simulink model "Crane_rigid"  (R2021b)
settings: Solver=ode15s  StartTime=0.0  StopTime=t_f  MaxStep=max_step_size  RelTol=1e-3
values from neighbouring files (symbols this model uses):
  a_d_full_y = circshift(a_d_full_x,floor(1/h))/2    [modify_tracking.m]
  cont_param_10 = in    [double_pendulum.m]    (also in optimize_10_SMC_single_first_explicit.m = cont_param_10_surrogateopt)
  cont_param_11 = in    [double_pendulum.m]    (also in optimize_11_SMC_single_first_implicit.m = cont_param_11_surrogateopt)
  cont_param_12 = in    [double_pendulum.m]    (also in optimize_12_SMC_single_last_explicit.m = cont_param_12_surrogateopt)
  cont_param_13 = in    [double_pendulum.m]    (also in optimize_13_SMC_single_last_implicit.m = cont_param_13_surrogateopt)
  cont_param_14 = in    [double_pendulum.m]    (also in optimize_14_SMC_double_explicit.m = cont_param_14_surrogateopt)
  cont_param_15 = in    [double_pendulum.m]    (also in optimize_15_SMC_double_implicit.m = cont_param_15_surrogateopt)
  cont_param_16 = in    [double_pendulum.m]
  cont_param_17 = in    [double_pendulum.m]
  cont_param_18 = in    [double_pendulum.m]
  cont_param_19 = in    [double_pendulum.m]
  cont_param_4 = in    [double_pendulum.m]
  cont_param_5 = in    [double_pendulum.m]
  cont_param_6 = in    [double_pendulum.m]
  cont_param_7 = in    [double_pendulum.m]
  cont_param_8 = in    [double_pendulum.m]
  cont_param_9 = in    [double_pendulum.m]
  h = 1e-5    (= 1e-05)    [Conference_paper.m]    (also in Latest.m)
  m = 10    [Conference_paper.m]    (also in Latest.m = 100; control_8_collocated_PD_tracking.m = load_mass+hook_mass+cable_mass_total)
  method_select = Method    [main_run.m]    (also in modify_tracking.m = 3)
  N = floor(t_f / h)    [control_2_zero_vibration.m]    (also in control_3_ZVD.m; modify_tracking.m = 3)
  s = c1*(x-xd)+c2*(v-vd)+c3*theta_dot_1+c4*theta_1    [control_10_SMC_single_first_explicit.m]    (also in control_11_SMC_single_first_implicit.m = c1*(x-xd)+c2*(v-vd)+c3*theta_dot+c4*theta; control_12_SMC_single_last_explicit.m = c1*(x-xd)+c2*(v-vd)+c3*theta_dot_2+c4*theta_2; control_13_SMC_single_last_implicit.m = c1*(x-xd)+c2*(v-vd)+c3*theta_dot+c4*theta; control_14_SMC_double_explicit.m = (v-vd)+lambda*(x-xd)+alpha*theta_1+beta*theta_2)
  sin_traj_w = 0.5    [modify_tracking.m]
  X = ex+lambda*sin(theta)    [control_16_PD_energy_first.m]    (also in control_17_PD_energy_last.m)
  Z = cont_param_8(4)    [control_8_collocated_PD_tracking.m]
undefined symbols (not defined in the file or in its folder): a_d_full_x, all_initial_sway, c_actuator, cable_length, cable_mass_total, cart_disturbance_amp, cart_mass, delay_time, first_link_sway, hook_mass, last_piece_length, load_disturbance_amp, number_of_pendulums, payload_mass, sat_const, sin_traj_A, t_f, total_mass, traj_number, unbalanced_factor, Y
libraries: nesl_utility x180, sm_lib x138, commchan3 x8
(part 1 of 3)
settings Model: Creator=rmoja  LastModifiedBy=SESA642626

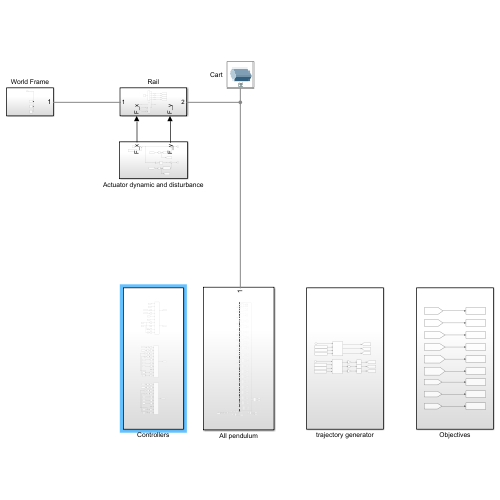
[thumbnail: Simulink's stored preview of the top-level diagram]
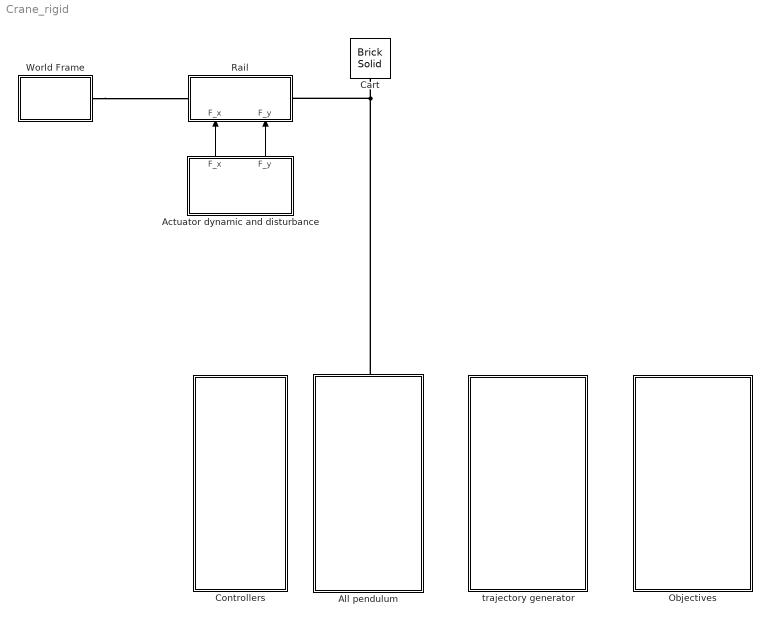
== system Crane_rigid ==
  Actuator dynamic and disturbance : Subsystem
  All pendulum : Subsystem
      settings: PortSchema="{\"entries\":[{\"content\":{\"sides\":[{\"content\":{\"connectorIds\":[]},\"type\":\"ConnectorPlacement.EquallySpacedRectSide\",\"uuid\":\"a0695cec-8b60-4481-8da3-91054655feca\"},{\"content\":{\"connectorIds\":[],\"side\":\"RIGHT\"},\"type\":\"ConnectorPlacement.EquallySpacedRectSide\",\"uuid\":\"63fc90b5-61bb-43b2-b1de-87e85d16d1ba\"},{\"content\":{\"connectorIds\":[\"LConn1\"],\"side\":\"TOP\"},\"type\":\"ConnectorPlacement.EquallySpacedRectSide\",\"uuid\":\"b1a79959-5d9b-4237-a357-9ee6cf3ddb2d\"}]},\"type\":\"ConnectorPlacement.EquallySpacedConnector\",\"uuid\":\"2998d234-7b55-409a-8879-2241677dc568\"}],\"packageUris\":[\"http://schema.mathworks.com/mf0/Connector/R2020b\"],\"version\":\"1.0\"}"
  Cart : sm_lib/Body Elements/Brick Solid  GraphicAmbientColor=[0.15 0.15 0.15 1.0]  BasedOnType=Mass  BrickDimensions=[1 1 1]  BrickDimensionUnits=m  CenterOfMass=[0 0 0]  CenterOfMassUnits=m  GraphicDiffuseColor=[0.8 0.0 0.8]  Density=1000  DensityUnits=kg/(m^3)  DoExposeReferenceFrame=on  GraphicEmissiveColor=[0.0 0.0 0.0 1.0]  ExportEntireGeometry=off  SerializedFrames=<Frames/>  MarkerShape=Sphere  MarkerSize=10  GraphicType=FromGeometry  InertiaType=PointMass  Mass=cart_mass  MassUnits=kg  MomentsOfInertia=[1 1 1]  MomentsOfInertiaUnits=kg*m^2  GraphicOpacity=1.0  ProductsOfInertia=[0 0 0]  ProductsOfInertiaUnits=kg*m^2  GraphicShininess=75  GraphicSpecularColor=[0.5 0.5 0.5 1.0]  GraphicVisPropType=SimpleVisualProperties
  Controllers : Subsystem
  Objectives : Subsystem
  Rail : Subsystem
      settings: PortSchema="{\"entries\":[{\"content\":{\"sides\":[{\"content\":{\"connectorIds\":[\"LConn1\"]},\"type\":\"ConnectorPlacement.EquallySpacedRectSide\",\"uuid\":\"d9e65a69-c05e-4610-81fe-2f9f88514456\"},{\"content\":{\"connectorIds\":[\"RConn1\"],\"side\":\"RIGHT\"},\"type\":\"ConnectorPlacement.EquallySpacedRectSide\",\"uuid\":\"de9124b5-abd7-4a44-8ac0-9f1bb82b9c20\"},{\"content\":{\"connectorIds\":[],\"side\":\"TOP\"},\"type\":\"ConnectorPlacement.EquallySpacedRectSide\",\"uuid\":\"433c8926-32eb-4eac-9405-2f674875eeab\"},{\"content\":{\"connectorIds\":[\"In1\",\"In2\"],\"side\":\"BOTTOM\"},\"type\":\"ConnectorPlacement.EquallySpacedRectSide\",\"uuid\":\"d2188721-54bd-44ea-91c1-f694293db46f\"}]},\"type\":\"ConnectorPlacement.EquallySpacedConnector\",\"uuid\":\"441db2e5-934f-48d0-8bd6-b56c902c81c4\"}],\"packageUris\":[\"http://schema.mathworks.com/mf0/Connector/R2020b\"],\"version\":\"1.0\"}"
  World Frame : Subsystem
  trajectory generator : Subsystem
  wires:
  Actuator dynamic and disturbance/1(F_x) -> Rail/1(F_x)
  Actuator dynamic and disturbance/2(F_y) -> Rail/2(F_y)
  connections:
  World Frame/LConn1 -- Rail/LConn1
  All pendulum/LConn1 -- Rail/RConn1 -- Cart/RConn1

== system Crane_rigid/Actuator dynamic and disturbance ==
  Actuator : TransferFcn  Numerator=[c_actuator]  Denominator=[1 c_actuator]
  Actuator1 : TransferFcn  Numerator=[c_actuator]  Denominator=[1 c_actuator]
  Constant : Constant  Value=cart_disturbance_amp
  Gain : Gain  Gain=0.5
  Pulse Generator : DiscretePulseGenerator  PulseType=Time based  Amplitude=2*cart_disturbance_amp  Period=20  PulseWidth=50
  Saturation1 : Saturate  UpperLimit=+sat_const  LowerLimit=-sat_const
  Saturation2 : Saturate  UpperLimit=+sat_const  LowerLimit=-sat_const
  Sum : Sum  Inputs=|+-
  Sum1 : Sum  Inputs=|++
  Sum3 : Sum  Inputs=|++
  Transport Delay : TransportDelay
  F_x : Outport
  F_y : Outport  Port=2
  tag scope: F_x_after_sat=global, F_y_after_sat=global
  wires:
  Actuator/1 -> Sum1/2
  Sum1/1 -> F_x/1
  Saturation1/1 -> [F_x_after_sat], Actuator/1
  [Control_output_x] -> Saturation1/1
  Sum3/1 -> F_y/1
  [Control_output_y] -> Saturation2/1
  Saturation2/1 -> [F_y_after_sat], Actuator1/1
  Actuator1/1 -> Sum3/2
  Pulse Generator/1 -> Sum/1
  Constant/1 -> Sum/2
  Sum/1 -> Gain/1, Sum1/1
  Gain/1 -> Transport Delay/1
  Transport Delay/1 -> Sum3/1  "yd"

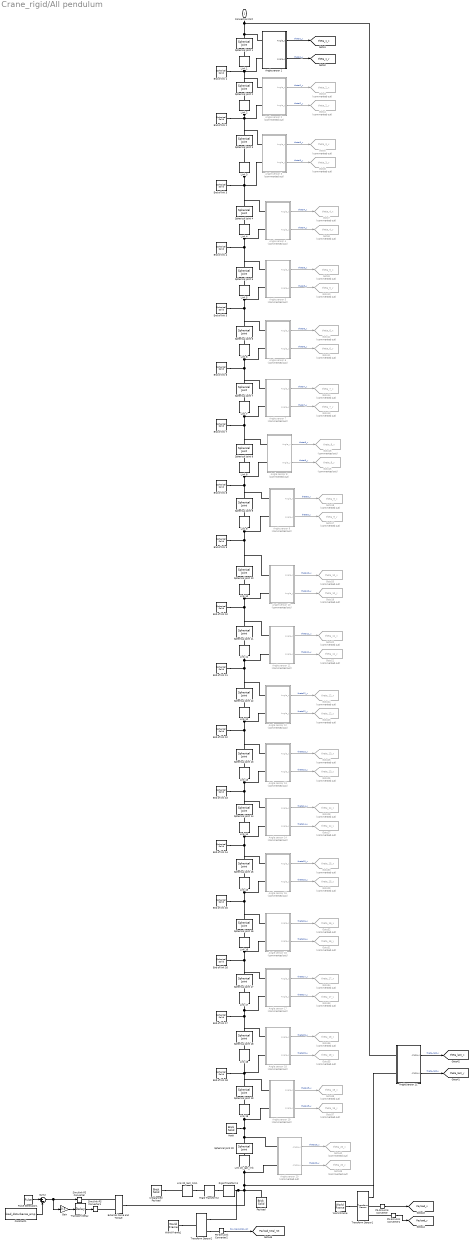
== system Crane_rigid/All pendulum ==
  Angle sensor 1 : Subsystem
  Angle sensor 10 : Subsystem  Commented=on
  Angle sensor 11 : Subsystem  Commented=on
  Angle sensor 12 : Subsystem  Commented=on
  Angle sensor 13 : Subsystem  Commented=on
  Angle sensor 14 : Subsystem  Commented=on
  Angle sensor 15 : Subsystem  Commented=on
  Angle sensor 16 : Subsystem  Commented=on
  Angle sensor 17 : Subsystem  Commented=on
  Angle sensor 18 : Subsystem  Commented=on
  Angle sensor 19 : Subsystem  Commented=on
  Angle sensor 2 : Subsystem  Commented=on
  Angle sensor 20 : Subsystem  Commented=on
  Angle sensor 21 : Subsystem
  Angle sensor 3 : Subsystem  Commented=on
  Angle sensor 4 : Subsystem  Commented=on
  Angle sensor 5 : Subsystem  Commented=on
  Angle sensor 6 : Subsystem  Commented=on
  Angle sensor 7 : Subsystem  Commented=on
  Angle sensor 8 : Subsystem  Commented=on
  Angle sensor 9 : Subsystem  Commented=on
  Constant1 : Constant  Value=load_disturbance_amp
  End of link {1..18} (18 alike) : sm_lib/Body Elements/Spherical Solid  GraphicAmbientColor=[0.15 0.15 0.15 1.0]  BasedOnType=Density  CenterOfMass=[0 0 0]  CenterOfMassUnits=m  GraphicDiffuseColor=[1.0 0.2 0.0]  Density=1000  DensityUnits=kg/(m^3)  DoExposeReferenceFrame=on  GraphicEmissiveColor=[0.0 0.0 0.0 1.0]  ExportEntireGeometry=off  SerializedExposedGeometries=<ExposedGeometries/>  SerializedFrames=<Frames/>  MarkerShape=Sphere  MarkerSize=10  GraphicType=FromGeometry  InertiaType=PointMass  Mass=0  MassUnits=kg  MomentsOfInertia=[1 1 1]*1e-3  MomentsOfInertiaUnits=kg*m^2  GraphicOpacity=1.0  ProductsOfInertia=[0 0 0]  ProductsOfInertiaUnits=kg*m^2  GraphicShininess=75  GraphicSpecularColor=[0.5 0.5 0.5 1.0]  SphereRadius=0.05  SphereRadiusUnits=m  GraphicVisPropType=SimpleVisualProperties
  External Force and Torque : sm_lib/Forces and Torques/External Force and Torque  ForceResolutionFrame=World  EnableForceX=on  EnableForceY=on  EnableForceZ=off  EnableForce=off  TorqueResolutionFrame=AttachedFrame  EnableTorqueX=off  EnableTorqueY=off  EnableTorqueZ=off  EnableTorque=off
  Gain : Gain  Gain=0.5
  Goto10 : Goto  Commented=on  GotoTag=theta_5_y  TagVisibility=global
  Goto11 : Goto  Commented=on  GotoTag=theta_6_y  TagVisibility=global
  Goto12 : Goto  Commented=on  GotoTag=theta_6_x  TagVisibility=global
  Goto13 : Goto  Commented=on  GotoTag=theta_7_y  TagVisibility=global
  Goto14 : Goto  Commented=on  GotoTag=theta_7_x  TagVisibility=global
  Goto15 : Goto  Commented=on  GotoTag=theta_8_y  TagVisibility=global
  Goto16 : Goto  Commented=on  GotoTag=theta_8_x  TagVisibility=global
  Goto17 : Goto  Commented=on  GotoTag=theta_9_y  TagVisibility=global
  Goto18 : Goto  Commented=on  GotoTag=theta_9_x  TagVisibility=global
  Goto19 : Goto  Commented=on  GotoTag=theta_10_y  TagVisibility=global
  Goto20 : Goto  Commented=on  GotoTag=theta_10_x  TagVisibility=global
  Goto21 : Goto  Commented=on  GotoTag=theta_11_y  TagVisibility=global
  Goto22 : Goto  Commented=on  GotoTag=theta_11_x  TagVisibility=global
  Goto23 : Goto  Commented=on  GotoTag=theta_12_y  TagVisibility=global
  Goto24 : Goto  Commented=on  GotoTag=theta_12_x  TagVisibility=global
  Goto25 : Goto  Commented=on  GotoTag=theta_13_y  TagVisibility=global
  Goto26 : Goto  Commented=on  GotoTag=theta_13_x  TagVisibility=global
  Goto27 : Goto  Commented=on  GotoTag=theta_14_y  TagVisibility=global
  Goto28 : Goto  Commented=on  GotoTag=theta_14_x  TagVisibility=global
  Goto29 : Goto  Commented=on  GotoTag=theta_15_y  TagVisibility=global
  Goto3 : Goto  Commented=on  GotoTag=theta_2_x  TagVisibility=global
  Goto30 : Goto  Commented=on  GotoTag=theta_15_x  TagVisibility=global
  Goto31 : Goto  Commented=on  GotoTag=theta_16_y  TagVisibility=global
  Goto32 : Goto  Commented=on  GotoTag=theta_16_x  TagVisibility=global
  Goto33 : Goto  Commented=on  GotoTag=theta_17_y  TagVisibility=global
  Goto34 : Goto  Commented=on  GotoTag=theta_17_x  TagVisibility=global
  Goto35 : Goto  Commented=on  GotoTag=theta_18_y  TagVisibility=global
  Goto36 : Goto  Commented=on  GotoTag=theta_18_x  TagVisibility=global
  Goto37 : Goto  Commented=on  GotoTag=theta_19_y  TagVisibility=global
  Goto38 : Goto  Commented=on  GotoTag=theta_19_x  TagVisibility=global
  Goto39 : Goto  Commented=on  GotoTag=theta_20_y  TagVisibility=global
  Goto4 : Goto  Commented=on  GotoTag=theta_2_y  TagVisibility=global
  Goto40 : Goto  Commented=on  GotoTag=theta_20_x  TagVisibility=global
  Goto5 : Goto  Commented=on  GotoTag=theta_3_x  TagVisibility=global
  Goto6 : Goto  Commented=on  GotoTag=theta_3_y  TagVisibility=global
  Goto7 : Goto  Commented=on  GotoTag=theta_4_x  TagVisibility=global
  Goto8 : Goto  Commented=on  GotoTag=theta_4_y  TagVisibility=global
  Goto9 : Goto  Commented=on  GotoTag=theta_5_x  TagVisibility=global
  Hook : sm_lib/Body Elements/Brick Solid  GraphicAmbientColor=[0.15 0.15 0.15 1.0]  BasedOnType=Mass  BrickDimensions=[0.2 0.2 0.1]  BrickDimensionUnits=m  CenterOfMass=[0 0 0]  CenterOfMassUnits=m  GraphicDiffuseColor=[0.2 0.6 0.0]  Density=1000  DensityUnits=kg/(m^3)  DoExposeReferenceFrame=on  GraphicEmissiveColor=[0.0 0.0 0.0 1.0]  ExportEntireGeometry=off  SerializedFrames=<Frames/>  MarkerShape=Sphere  MarkerSize=10  GraphicType=FromGeometry  InertiaType=CalculateFromGeometry  Mass=hook_mass  MassUnits=kg  MomentsOfInertia=[1 1 1]  MomentsOfInertiaUnits=kg*m^2  GraphicOpacity=1.0  ProductsOfInertia=[0 0 0]  ProductsOfInertiaUnits=kg*m^2  GraphicShininess=75  GraphicSpecularColor=[0.5 0.5 0.5 1.0]  GraphicVisPropType=SimpleVisualProperties
  Link {1..19} (19 alike) : sm_lib/Body Elements/Cylindrical Solid  GraphicAmbientColor=[0.15 0.15 0.15 1.0]  BasedOnType=Density  CenterOfMass=[0 0 0]  CenterOfMassUnits=m  GraphicDiffuseColor=[0.5 0.5 0.5]  CylinderLength=cable_length/number_of_pendulums  CylinderLengthUnits=m  CylinderRadius=0.02  CylinderRadiusUnits=m  Density=1000  DensityUnits=kg/m^3  DoExposeReferenceFrame=off  GraphicEmissiveColor=[0.0 0.0 0.0 1.0]  ExportEntireGeometry=off  SerializedFrames=<Frames><Frame><Id>Frame1</Id><Value><Name>F1</Name><Origin><Source>GeometricFeature</Source><FeatureName>top surface</FeatureName></Origin><PrimaryAxis><DefinedDirection>+Z</DefinedDirection><Source>ReferenceFrame</Source><SourceDirection>+Z</SourceDirection><FeatureName></FeatureName></PrimaryAxis><SecondaryAxis><DefinedDirection>+X</DefinedDirection><Source>ReferenceFrame</Source><SourceDirection>+X</SourceDirection><FeatureName></FeatureName></SecondaryAxis></Value></Frame><Frame><Id>Frame2</Id><Value><Name>F2</Name><Origin><Source>GeometricFeature</Source><FeatureName>bottom curve</FeatureName></Origin><PrimaryAxis><DefinedDirection>+Z</DefinedDirection><Source>ReferenceFrame</Source><SourceDirection>+Z</SourceDirection><FeatureName></FeatureName></PrimaryAxis><SecondaryAxis><DefinedDirection>+X</DefinedDirection><Source>ReferenceFrame</Source><SourceDirection>+X</SourceDirection><FeatureName></FeatureName></SecondaryAxis></Value></Frame></Frames>  MarkerShape=Sphere  MarkerSize=10  GraphicType=FromGeometry  InertiaType=CalculateFromGeometry  Mass=1  MassUnits=kg  MomentsOfInertia=[1 1 1]  MomentsOfInertiaUnits=kg*m^2  GraphicOpacity=1.0  ProductsOfInertia=[0 0 0]  ProductsOfInertiaUnits=kg*m^2  GraphicShininess=75  GraphicSpecularColor=[0.5 0.5 0.5 1.0]  GraphicVisPropType=SimpleVisualProperties
  Link 20_last_link : sm_lib/Body Elements/Cylindrical Solid  GraphicAmbientColor=[0.15 0.15 0.15 1.0]  BasedOnType=Density  CenterOfMass=[0 0 0]  CenterOfMassUnits=m  GraphicDiffuseColor=[0.5 0.5 0.5]  CylinderLength=last_piece_length  CylinderLengthUnits=m  CylinderRadius=0.02  CylinderRadiusUnits=m  Density=1000  DensityUnits=kg/m^3  DoExposeReferenceFrame=off  GraphicEmissiveColor=[0.0 0.0 0.0 1.0]  ExportEntireGeometry=off  SerializedFrames=<Frames><Frame><Id>Frame1</Id><Value><Name>F1</Name><Origin><Source>GeometricFeature</Source><FeatureName>top surface</FeatureName></Origin><PrimaryAxis><DefinedDirection>+Z</DefinedDirection><Source>ReferenceFrame</Source><SourceDirection>+Z</SourceDirection><FeatureName></FeatureName></PrimaryAxis><SecondaryAxis><DefinedDirection>+X</DefinedDirection><Source>ReferenceFrame</Source><SourceDirection>+X</SourceDirection><FeatureName></FeatureName></SecondaryAxis></Value></Frame><Frame><Id>Frame2</Id><Value><Name>F2</Name><Origin><Source>GeometricFeature</Source><FeatureName>bottom curve</FeatureName></Origin><PrimaryAxis><DefinedDirection>+Z</DefinedDirection><Source>ReferenceFrame</Source><SourceDirection>+Z</SourceDirection><FeatureName></FeatureName></PrimaryAxis><SecondaryAxis><DefinedDirection>+X</DefinedDirection><Source>ReferenceFrame</Source><SourceDirection>+X</SourceDirection><FeatureName></FeatureName></SecondaryAxis></Value></Frame></Frames>  MarkerShape=Sphere  MarkerSize=10  GraphicType=FromGeometry  InertiaType=CalculateFromGeometry  Mass=1  MassUnits=kg  MomentsOfInertia=[1 1 1]  MomentsOfInertiaUnits=kg*m^2  GraphicOpacity=1.0  ProductsOfInertia=[0 0 0]  ProductsOfInertiaUnits=kg*m^2  GraphicShininess=75  GraphicSpecularColor=[0.5 0.5 0.5 1.0]  GraphicVisPropType=SimpleVisualProperties
  Link 20_last_link1 : sm_lib/Body Elements/Cylindrical Solid  GraphicAmbientColor=[0.15 0.15 0.15 1.0]  BasedOnType=Mass  CenterOfMass=[0 0 0]  CenterOfMassUnits=m  GraphicDiffuseColor=[0.6 0.0 0.6]  CylinderLength=1  CylinderLengthUnits=m  CylinderRadius=0.05  CylinderRadiusUnits=m  Density=1000  DensityUnits=kg/m^3  DoExposeReferenceFrame=off  GraphicEmissiveColor=[0.0 0.0 0.0 1.0]  ExportEntireGeometry=off  SerializedFrames=<Frames><Frame><Id>Frame1</Id><Value><Name>F1</Name><Origin><Source>GeometricFeature</Source><FeatureName>top surface</FeatureName></Origin><PrimaryAxis><DefinedDirection>+Z</DefinedDirection><Source>ReferenceFrame</Source><SourceDirection>+Z</SourceDirection><FeatureName></FeatureName></PrimaryAxis><SecondaryAxis><DefinedDirection>+X</DefinedDirection><Source>ReferenceFrame</Source><SourceDirection>+X</SourceDirection><FeatureName></FeatureName></SecondaryAxis></Value></Frame><Frame><Id>Frame2</Id><Value><Name>F2</Name><Origin><Source>GeometricFeature</Source><FeatureName>bottom curve</FeatureName></Origin><PrimaryAxis><DefinedDirection>+Z</DefinedDirection><Source>ReferenceFrame</Source><SourceDirection>+Z</SourceDirection><FeatureName></FeatureName></PrimaryAxis><SecondaryAxis><DefinedDirection>+X</DefinedDirection><Source>ReferenceFrame</Source><SourceDirection>+X</SourceDirection><FeatureName></FeatureName></SecondaryAxis></Value></Frame></Frames>  MarkerShape=Sphere  MarkerSize=10  GraphicType=FromGeometry  InertiaType=CalculateFromGeometry  Mass=0  MassUnits=kg  MomentsOfInertia=[1 1 1]  MomentsOfInertiaUnits=kg*m^2  GraphicOpacity=1.0  ProductsOfInertia=[0 0 0]  ProductsOfInertiaUnits=kg*m^2  GraphicShininess=75  GraphicSpecularColor=[0.5 0.5 0.5 1.0]  GraphicVisPropType=SimpleVisualProperties
  PS-Simulink Converter : nesl_utility/PS-Simulink Converter  PhysicalDomain=network_engine_domain  SubClassName=ps_output  LeftPortType=input  RightPortType=output  PseudoPeriodic=off  Frequencies=[]  Unit=inherit  AffineConversion=off
      settings: SourceProductBaseCode=PW,SS
  PS-Simulink Converter1 : nesl_utility/PS-Simulink Converter  PhysicalDomain=network_engine_domain  SubClassName=ps_output  LeftPortType=input  RightPortType=output  PseudoPeriodic=off  Frequencies=[]  Unit=inherit  AffineConversion=off
      settings: SourceProductBaseCode=PW,SS
  PS-Simulink Converter2 : nesl_utility/PS-Simulink Converter  PhysicalDomain=network_engine_domain  SubClassName=ps_output  LeftPortType=input  RightPortType=output  PseudoPeriodic=off  Frequencies=[]  Unit=inherit  AffineConversion=off
      settings: SourceProductBaseCode=PW,SS
  Payload : sm_lib/Body Elements/Brick Solid  GraphicAmbientColor=[0.15 0.15 0.15 1.0]  BasedOnType=Mass  BrickDimensions=[1 1 0.5]  BrickDimensionUnits=m  CenterOfMass=[0 0 0]  CenterOfMassUnits=m  GraphicDiffuseColor=[0 0 1]  Density=1000  DensityUnits=kg/(m^3)  DoExposeReferenceFrame=on  GraphicEmissiveColor=[0.0 0.0 0.0 1.0]  ExportEntireGeometry=off  SerializedFrames=<Frames/>  MarkerShape=Sphere  MarkerSize=10  GraphicType=FromGeometry  InertiaType=CalculateFromGeometry  Mass=payload_mass*(1-unbalanced_factor)  MassUnits=kg  MomentsOfInertia=[1 1 1]  MomentsOfInertiaUnits=kg*m^2  GraphicOpacity=1.0  ProductsOfInertia=[0 0 0]  ProductsOfInertiaUnits=kg*m^2  GraphicShininess=75  GraphicSpecularColor=[0.5 0.5 0.5 1.0]  GraphicVisPropType=SimpleVisualProperties
  Pulse Generator1 : DiscretePulseGenerator  PulseType=Time based  Amplitude=2*load_disturbance_amp  Period=20  PulseWidth=50
  Rigid Transform1 : sm_lib/Frames and Transforms/Rigid Transform  TranslationMethod=Cartesian  TranslationStandardOffset=0  TranslationLengthUnit=m  TranslationStandardAxis=+Z  TranslationCartesianOffset=[0 0 0]  TranslationROffset=0  TranslationROffsetUnits=m  TranslationZOffset=0  TranslationZOffsetUnits=m  TranslationThetaOffset=0  TranslationThetaOffsetUnits=deg  RotationMethod=StandardAxis  RotationAngleUnits=deg  RotationStandardAxis=+Y  RotationAngle=90  RotationArbitraryAxis=[0 0 1]  FollAlignAxisA=+X  BaseAlignAxisA=+Y  FollAlignAxisB=+Y  BaseAlignAxisB=+Z  RotationSequenceAxes=FollowerAxes  RotationSequence=XYX  RotationSequenceAngles=[0 0 0]  RotationSequenceAnglesUnits=deg  RotationMatrix=[1 0 0; 0 1 0; 0 0 1]
  Rigid Transform2 : sm_lib/Frames and Transforms/Rigid Transform  TranslationMethod=Cartesian  TranslationStandardOffset=0  TranslationLengthUnit=m  TranslationStandardAxis=+Z  TranslationCartesianOffset=[0 0 0]  TranslationROffset=0  TranslationROffsetUnits=m  TranslationZOffset=0  TranslationZOffsetUnits=m  TranslationThetaOffset=0  TranslationThetaOffsetUnits=deg  RotationMethod=StandardAxis  RotationAngleUnits=deg  RotationStandardAxis=+X  RotationAngle=90  RotationArbitraryAxis=[0 0 1]  FollAlignAxisA=+X  BaseAlignAxisA=+Y  FollAlignAxisB=+Y  BaseAlignAxisB=+Z  RotationSequenceAxes=FollowerAxes  RotationSequence=XYX  RotationSequenceAngles=[0 0 0]  RotationSequenceAnglesUnits=deg  RotationMatrix=[1 0 0; 0 1 0; 0 0 1]
  Simulink-PS Converter : nesl_utility/Simulink-PS Converter  PhysicalDomain=network_engine_domain  SubClassName=ps_input  LeftPortType=input  RightPortType=output  PseudoPeriodic=off  Frequencies=[]  NoiseDistribution=none  NoiseParameters=[]  Unit=1  AffineConversion=off  FilteringAndDerivatives=provide  SimscapeFilterOrder=1  InputFilterTimeConstant=0.001  UdotUserProvided=0
      settings: SourceProductBaseCode=PW,SS
  Simulink-PS Converter1 : nesl_utility/Simulink-PS Converter  PhysicalDomain=network_engine_domain  SubClassName=ps_input  LeftPortType=input  RightPortType=output  PseudoPeriodic=off  Frequencies=[]  NoiseDistribution=none  NoiseParameters=[]  Unit=1  AffineConversion=off  FilteringAndDerivatives=provide  SimscapeFilterOrder=1  InputFilterTimeConstant=0.001  UdotUserProvided=0
      settings: SourceProductBaseCode=PW,SS
  Spherical Joint 1 : sm_lib/Joints/Spherical Joint  JointMode=Normal  SenseConstraintForce=off  SenseConstraintForceX=off  SenseConstraintForceY=off  SenseConstraintForceZ=off  SenseConstraintTorque=off  SenseConstraintTorqueX=off  SenseConstraintTorqueY=off  SenseConstraintTorqueZ=off  SenseTotalForce=off  SenseTotalForceX=off  SenseTotalForceY=off  SenseTotalForceZ=off  SenseTotalTorque=off  SenseTotalTorqueX=off  SenseTotalTorqueY=off  SenseTotalTorqueZ=off  CompositeWrenchDir=FollowerOnBase  CompositeWrenchFrame=BaseFrame  DefPosRotationMethod=None  DefPosRotationAngleUnits=deg  DefPosRotationStandardAxis=+Z  DefPosRotationAngle=0.0  DefPosRotationArbitraryAxis=[0 0 1]  DefPosFollAlignAxisA=+X  DefPosBaseAlignAxisA=+Y  DefPosFollAlignAxisB=+Y  DefPosBaseAlignAxisB=+Z  DefPosRotationSequenceAxes=FollowerAxes  DefPosRotationSequence=XYX  DefPosRotationSequenceAngles=[0 0 0]  DefPosRotationSequenceAnglesUnits=deg  DefPosRotationMatrix=[1 0 0; 0 1 0; 0 0 1]  EqPosRotationMethod=None  EqPosRotationAngleUnits=deg  EqPosRotationStandardAxis=+Z  EqPosRotationAngle=0.0  EqPosRotationArbitraryAxis=[0 0 1]  EqPosFollAlignAxisA=+X  EqPosBaseAlignAxisA=+Y  EqPosFollAlignAxisB=+Y  EqPosBaseAlignAxisB=+Z  EqPosRotationSequenceAxes=FollowerAxes  EqPosRotationSequence=XYX  EqPosRotationSequenceAngles=[0 0 0]  EqPosRotationSequenceAnglesUnits=deg  EqPosRotationMatrix=[1 0 0; 0 1 0; 0 0 1]  SpringStiffness=joint_stiffness  SpringStiffnessUnits=N*m/deg  DampingCoefficient=damping_coefficient  DampingCoefficientUnits=N*m/(deg/s)  ActuateTorqueX=off  ActuateTorqueY=off  ActuateTorqueZ=off  ActuateTorque=off  TorqueActuationMode=NoTorque  MotionActuationMode=ComputedMotion  ActuationFrame=BaseFrame  SensePosition=off  SenseVelocityX=off  SenseVelocityY=off  SenseVelocityZ=off  SenseVelocity=off  SenseAccelerationX=off  SenseAccelerationY=off  SenseAccelerationZ=off  SenseAcceleration=off  SenseTorqueX=off  SenseTorqueY=off  SenseTorqueZ=off  SenseTorqueForce=off  SenseLowerLimitTorqueMag=off  SenseUpperLimitTorqueMag=off  SensingFrame=BaseFrame  LowerLimitSpecify=off  LowerLimitBound=15  LowerLimitBoundUnits=deg  LowerLimitStiffness=1e4  LowerLimitStiffnessUnits=N*m/deg  LowerLimitDamping=10  LowerLimitDampingUnits=N*m/(deg/s)  LowerLimitTransitionRegionWidth=0.1  LowerLimitTransitionRegionWidthUnits=deg  UpperLimitSpecify=off  UpperLimitBound=45  UpperLimitBoundUnits=deg  UpperLimitStiffness=1e4  UpperLimitStiffnessUnits=N*m/deg  UpperLimitDamping=10  UpperLimitDampingUnits=N*m/(deg/s)  UpperLimitTransitionRegionWidth=0.1  UpperLimitTransitionRegionWidthUnits=deg  PositionTargetRotationMethod=StandardAxis  PositionTargetRotationAngleUnits=deg  PositionTargetRotationStandardAxis=+Y  PositionTargetRotationAngle=first_link_sway+all_initial_sway  PositionTargetRotationArbitraryAxis=[1 1 1]  PositionTargetFollAlignAxisA=+X  PositionTargetBaseAlignAxisA=-Z  PositionTargetFollAlignAxisB=+Y  PositionTargetBaseAlignAxisB=-Z  PositionTargetRotationSequenceAxes=BaseAxes  PositionTargetRotationSequence=XYX  PositionTargetRotationSequenceAngles=[15 0 0]  PositionTargetRotationSequenceAnglesUnits=deg  PositionTargetRotationMatrix=[1 0 0; 0 1 0; 0 0 1]  PositionTargetSpecify=on  PositionTargetPriority=High  VelocityTargetValue=[0 0 0]  VelocityTargetValueUnits=deg/s  VelocityTargetSpecify=off  VelocityTargetPriority=High  VelocityTargetInFollowerFrame=on
  Spherical Joint {2..20} (19 alike) : sm_lib/Joints/Spherical Joint  JointMode=Normal  SenseConstraintForce=off  SenseConstraintForceX=off  SenseConstraintForceY=off  SenseConstraintForceZ=off  SenseConstraintTorque=off  SenseConstraintTorqueX=off  SenseConstraintTorqueY=off  SenseConstraintTorqueZ=off  SenseTotalForce=off  SenseTotalForceX=off  SenseTotalForceY=off  SenseTotalForceZ=off  SenseTotalTorque=off  SenseTotalTorqueX=off  SenseTotalTorqueY=off  SenseTotalTorqueZ=off  CompositeWrenchDir=FollowerOnBase  CompositeWrenchFrame=BaseFrame  DefPosRotationMethod=None  DefPosRotationAngleUnits=deg  DefPosRotationStandardAxis=+Z  DefPosRotationAngle=0.0  DefPosRotationArbitraryAxis=[0 0 1]  DefPosFollAlignAxisA=+X  DefPosBaseAlignAxisA=+Y  DefPosFollAlignAxisB=+Y  DefPosBaseAlignAxisB=+Z  DefPosRotationSequenceAxes=FollowerAxes  DefPosRotationSequence=XYX  DefPosRotationSequenceAngles=[0 0 0]  DefPosRotationSequenceAnglesUnits=deg  DefPosRotationMatrix=[1 0 0; 0 1 0; 0 0 1]  EqPosRotationMethod=None  EqPosRotationAngleUnits=deg  EqPosRotationStandardAxis=+Z  EqPosRotationAngle=0.0  EqPosRotationArbitraryAxis=[0 0 1]  EqPosFollAlignAxisA=+X  EqPosBaseAlignAxisA=+Y  EqPosFollAlignAxisB=+Y  EqPosBaseAlignAxisB=+Z  EqPosRotationSequenceAxes=FollowerAxes  EqPosRotationSequence=XYX  EqPosRotationSequenceAngles=[0 0 0]  EqPosRotationSequenceAnglesUnits=deg  EqPosRotationMatrix=[1 0 0; 0 1 0; 0 0 1]  SpringStiffness=joint_stiffness  SpringStiffnessUnits=N*m/deg  DampingCoefficient=damping_coefficient  DampingCoefficientUnits=N*m/(deg/s)  ActuateTorqueX=off  ActuateTorqueY=off  ActuateTorqueZ=off  ActuateTorque=off  TorqueActuationMode=NoTorque  MotionActuationMode=ComputedMotion  ActuationFrame=BaseFrame  SensePosition=off  SenseVelocityX=off  SenseVelocityY=off  SenseVelocityZ=off  SenseVelocity=off  SenseAccelerationX=off  SenseAccelerationY=off  SenseAccelerationZ=off  SenseAcceleration=off  SenseTorqueX=off  SenseTorqueY=off  SenseTorqueZ=off  SenseTorqueForce=off  SenseLowerLimitTorqueMag=off  SenseUpperLimitTorqueMag=off  SensingFrame=BaseFrame  LowerLimitSpecify=off  LowerLimitBound=15  LowerLimitBoundUnits=deg  LowerLimitStiffness=1e4  LowerLimitStiffnessUnits=N*m/deg  LowerLimitDamping=10  LowerLimitDampingUnits=N*m/(deg/s)  LowerLimitTransitionRegionWidth=0.1  LowerLimitTransitionRegionWidthUnits=deg  UpperLimitSpecify=off  UpperLimitBound=45  UpperLimitBoundUnits=deg  UpperLimitStiffness=1e4  UpperLimitStiffnessUnits=N*m/deg  UpperLimitDamping=10  UpperLimitDampingUnits=N*m/(deg/s)  UpperLimitTransitionRegionWidth=0.1  UpperLimitTransitionRegionWidthUnits=deg  PositionTargetRotationMethod=StandardAxis  PositionTargetRotationAngleUnits=deg  PositionTargetRotationStandardAxis=+Y  PositionTargetRotationAngle=all_initial_sway  PositionTargetRotationArbitraryAxis=[1 1 1]  PositionTargetFollAlignAxisA=+X  PositionTargetBaseAlignAxisA=-Z  PositionTargetFollAlignAxisB=+Y  PositionTargetBaseAlignAxisB=-Z  PositionTargetRotationSequenceAxes=BaseAxes  PositionTargetRotationSequence=XYX  PositionTargetRotationSequenceAngles=[15 0 0]  PositionTargetRotationSequenceAnglesUnits=deg  PositionTargetRotationMatrix=[1 0 0; 0 1 0; 0 0 1]  PositionTargetSpecify=on  PositionTargetPriority=High  VelocityTargetValue=[0 0 0]  VelocityTargetValueUnits=deg/s  VelocityTargetSpecify=off  VelocityTargetPriority=High  VelocityTargetInFollowerFrame=on
  Sum2 : Sum  Inputs=|+-
  Transform Sensor1 : sm_lib/Frames and Transforms/Transform Sensor  MeasurementFrame=World  SenseAngle=off  SenseAxis=off  SenseAngle1=off  SenseAngle2=off  SenseAngle3=off  SenseQ=off  SenseR=off  SenseOmegaX=off  SenseOmegaY=off  SenseOmegaZ=off  SenseOmega1=off  SenseOmega2=off  SenseOmega3=off  SenseQDot=off  SenseRDot=off  SenseAlphaX=off  SenseAlphaY=off  SenseAlphaZ=off  SenseAlpha1=off  SenseAlpha2=off  SenseAlpha3=off  SenseQDDot=off  SenseRDDot=off  SenseX=on  SenseY=on  SenseZ=off  SenseRad=off  SenseAzim=off  SenseDist=off  SenseInc=off  SenseXDot=off  SenseYDot=off  SenseZDot=off  SenseRadDot=off  SenseAzimDot=off  SenseDistDot=off  SenseIncDot=off  SenseXDDot=off  SenseYDDot=off  SenseZDDot=off  SenseRadDDot=off  SenseAzimDDot=off  SenseDistDDot=off  SenseIncDDot=off
  Transform Sensor2 : sm_lib/Frames and Transforms/Transform Sensor  MeasurementFrame=World  SenseAngle=on  SenseAxis=off  SenseAngle1=off  SenseAngle2=off  SenseAngle3=off  SenseQ=off  SenseR=off  SenseOmegaX=off  SenseOmegaY=off  SenseOmegaZ=off  SenseOmega1=off  SenseOmega2=off  SenseOmega3=off  SenseQDot=off  SenseRDot=off  SenseAlphaX=off  SenseAlphaY=off  SenseAlphaZ=off  SenseAlpha1=off  SenseAlpha2=off  SenseAlpha3=off  SenseQDDot=off  SenseRDDot=off  SenseX=off  SenseY=off  SenseZ=off  SenseRad=off  SenseAzim=off  SenseDist=off  SenseInc=off  SenseXDot=off  SenseYDot=off  SenseZDot=off  SenseRadDot=off  SenseAzimDot=off  SenseDistDot=off  SenseIncDot=off  SenseXDDot=off  SenseYDDot=off  SenseZDDot=off  SenseRadDDot=off  SenseAzimDDot=off  SenseDistDDot=off  SenseIncDDot=off
  Transport Delay : TransportDelay
  Unbalanced Payload : sm_lib/Body Elements/Brick Solid  GraphicAmbientColor=[0.15 0.15 0.15 1.0]  BasedOnType=Mass  BrickDimensions=[0.2 0.2 0.1]  BrickDimensionUnits=m  CenterOfMass=[0 0 0]  CenterOfMassUnits=m  GraphicDiffuseColor=[0.0 0.8 0.2]  Density=1000  DensityUnits=kg/(m^3)  DoExposeReferenceFrame=on  GraphicEmissiveColor=[0.0 0.0 0.0 1.0]  ExportEntireGeometry=off  SerializedFrames=<Frames/>  MarkerShape=Sphere  MarkerSize=10  GraphicType=FromGeometry  InertiaType=PointMass  Mass=payload_mass*(unbalanced_factor)  MassUnits=kg  MomentsOfInertia=[1 1 1]  MomentsOfInertiaUnits=kg*m^2  GraphicOpacity=1.0  ProductsOfInertia=[0 0 0]  ProductsOfInertiaUnits=kg*m^2  GraphicShininess=75  GraphicSpecularColor=[0.5 0.5 0.5 1.0]  GraphicVisPropType=SimpleVisualProperties
  World Frame : sm_lib/Frames and Transforms/World Frame
  World Frame1 : sm_lib/Frames and Transforms/World Frame
  Connection Port : PMIOPort  Side=Left
  tag scope: Payload_total_rot=global, Payload_x=global, Payload_y=global, theta_1_x=global, theta_1_y=global, theta_last_x=global, theta_last_y=global
  wires:
  Angle sensor 1/1(Angle_x) -> [theta_1_x]  "theta1_x"
  Angle sensor 1/2(Angle_y) -> [theta_1_y]  "theta1_y"
  Angle sensor 2/2(Angle_y) -> Goto4/1  "theta2_y"
  Angle sensor 2/1(Angle_x) -> Goto3/1  "theta2_x"
  Angle sensor 3/2(Angle_y) -> Goto6/1  "theta3_y"
  Angle sensor 3/1(Angle_x) -> Goto5/1  "theta3_x"
  Angle sensor 4/1(Angle_x) -> Goto7/1  "theta4_x"
  Angle sensor 4/2(Angle_y) -> Goto8/1  "theta4_y"
  Angle sensor 5/2(Angle_y) -> Goto10/1  "theta5_y"
  Angle sensor 5/1(Angle_x) -> Goto9/1  "theta5_x"
  Angle sensor 6/1(Angle_x) -> Goto12/1  "theta6_x"
  Angle sensor 6/2(Angle_y) -> Goto11/1  "theta6_y"
  Angle sensor 7/2(Angle_y) -> Goto13/1  "theta7_y"
  Angle sensor 7/1(Angle_x) -> Goto14/1  "theta7_x"
  Angle sensor 8/1(Angle_x) -> Goto16/1  "theta8_x"
  Angle sensor 8/2(Angle_y) -> Goto15/1  "theta8_y"
  Angle sensor 9/2(Angle_y) -> Goto17/1  "theta9_y"
  Angle sensor 9/1(Angle_x) -> Goto18/1  "theta9_x"
  Angle sensor 10/1(Angle_x) -> Goto20/1  "theta10_x"
  Angle sensor 10/2(Angle_y) -> Goto19/1  "theta10_y"
  Angle sensor 11/2(Angle_y) -> Goto21/1  "theta11_y"
  Angle sensor 11/1(Angle_x) -> Goto22/1  "theta11_x"
  Angle sensor 12/1(Angle_x) -> Goto24/1  "theta12_x"
  Angle sensor 12/2(Angle_y) -> Goto23/1  "theta12_y"
  Angle sensor 13/2(Angle_y) -> Goto25/1  "theta13_y"
  Angle sensor 13/1(Angle_x) -> Goto26/1  "theta13_x"
  Angle sensor 14/1(Angle_x) -> Goto28/1  "theta14_x"
  Angle sensor 14/2(Angle_y) -> Goto27/1  "theta14_y"
  Angle sensor 15/2(Angle_y) -> Goto29/1  "theta15_y"
  Angle sensor 15/1(Angle_x) -> Goto30/1  "theta15_x"
  Angle sensor 16/1(Angle_x) -> Goto32/1  "theta16_x"
  Angle sensor 16/2(Angle_y) -> Goto31/1  "theta16_y"
  Angle sensor 17/2(Angle_y) -> Goto33/1  "theta17_y"
  Angle sensor 17/1(Angle_x) -> Goto34/1  "theta17_x"
  Angle sensor 18/1(Angle_x) -> Goto36/1  "theta18_x"
  Angle sensor 18/2(Angle_y) -> Goto35/1  "theta18_y"
  Angle sensor 19/2(Angle_y) -> Goto37/1  "theta19_y"
  Angle sensor 19/1(Angle_x) -> Goto38/1  "theta19_x"
  Angle sensor 20/1(Angle_x) -> Goto40/1  "theta20_x"
  Angle sensor 20/2(Angle_y) -> Goto39/1  "theta20_y"
  Angle sensor 21/1(Angle_x) -> [theta_last_x]  "theta_last_x"
  Angle sensor 21/2(Angle_y) -> [theta_last_y]  "theta_last_y"
  PS-Simulink Converter/1 -> [Payload_x]
  PS-Simulink Converter1/1 -> [Payload_y]
  PS-Simulink Converter2/1 -> [Payload_total_rot]  "Payload_total_rot"
  Constant1/1 -> Sum2/2
  Pulse Generator1/1 -> Sum2/1
  Sum2/1 -> Gain/1, Simulink-PS Converter/1
  Gain/1 -> Transport Delay/1
  Transport Delay/1 -> Simulink-PS Converter1/1
  connections:
  Angle sensor 8/LConn1 -- Spherical Joint 8/LConn1 -- End of link 7/RConn1 -- Angle sensor 7/LConn2 -- Link 7/RConn1
  Angle sensor 7/LConn1 -- Spherical Joint 7/LConn1 -- End of link 6/RConn1 -- Angle sensor 6/LConn2 -- Link 6/RConn1
  Link 1/RConn1 -- Angle sensor 2/LConn1 -- Spherical Joint 2/LConn1 -- Angle sensor 1/LConn2 -- End of link 1/RConn1
  End of link 8/RConn1 -- Angle sensor 9/LConn1 -- Spherical Joint 9/LConn1 -- Angle sensor 8/LConn2 -- Link 8/RConn1
  Angle sensor 5/LConn1 -- Spherical Joint 5/LConn1 -- End of link 4/RConn1 -- Angle sensor 4/LConn2 -- Link 4/RConn1
  Connection Port/RConn1 -- Angle sensor 1/LConn1 -- Spherical Joint 1/LConn1 -- Angle sensor 21/LConn1
  Link 2/RConn1 -- Angle sensor 3/LConn1 -- Spherical Joint 3/LConn1 -- End of link 2/RConn1 -- Angle sensor 2/LConn2
  End of link 9/RConn1 -- Angle sensor 10/LConn1 -- Spherical Joint 10/LConn1 -- Angle sensor 9/LConn2 -- Link 9/RConn1
  End of link 15/RConn1 -- Angle sensor 16/LConn1 -- Spherical Joint 16/LConn1 -- Angle sensor 15/LConn2 -- Link 15/RConn1
  End of link 17/RConn1 -- Angle sensor 18/LConn1 -- Spherical Joint 18/LConn1 -- Angle sensor 17/LConn2 -- Link 17/RConn1
  End of link 12/RConn1 -- Angle sensor 13/LConn1 -- Spherical Joint 13/LConn1 -- Angle sensor 12/LConn2 -- Link 12/RConn1
  End of link 16/RConn1 -- Angle sensor 17/LConn1 -- Spherical Joint 17/LConn1 -- Angle sensor 16/LConn2 -- Link 16/RConn1
  End of link 11/RConn1 -- Angle sensor 12/LConn1 -- Spherical Joint 12/LConn1 -- Angle sensor 11/LConn2 -- Link 11/RConn1
  End of link 10/RConn1 -- Angle sensor 11/LConn1 -- Spherical Joint 11/LConn1 -- Angle sensor 10/LConn2 -- Link 10/RConn1
  End of link 18/RConn1 -- Angle sensor 19/LConn1 -- Spherical Joint 19/LConn1 -- Angle sensor 18/LConn2 -- Link 18/RConn1
  Angle sensor 6/LConn1 -- Spherical Joint 6/LConn1 -- End of link 5/RConn1 -- Angle sensor 5/LConn2 -- Link 5/RConn1
  Link 3/RConn1 -- Angle sensor 4/LConn1 -- Spherical Joint 4/LConn1 -- Angle sensor 3/LConn2 -- End of link 3/RConn1
  Spherical Joint 20/LConn1 -- Angle sensor 20/LConn1 -- Hook/RConn1 -- Angle sensor 19/LConn2 -- Link 19/RConn1
  End of link 13/RConn1 -- Angle sensor 14/LConn1 -- Spherical Joint 14/LConn1 -- Angle sensor 13/LConn2 -- Link 13/RConn1
  End of link 14/RConn1 -- Angle sensor 15/LConn1 -- Spherical Joint 15/LConn1 -- Angle sensor 14/LConn2 -- Link 14/RConn1
  Link 10/LConn1 -- Spherical Joint 10/RConn1
  Link 19/LConn1 -- Spherical Joint 19/RConn1
  Link 3/LConn1 -- Spherical Joint 3/RConn1
  Link 20_last_link/LConn1 -- Spherical Joint 20/RConn1
  Link 9/LConn1 -- Spherical Joint 9/RConn1
  Link 15/LConn1 -- Spherical Joint 15/RConn1
  Link 6/LConn1 -- Spherical Joint 6/RConn1
  Link 14/LConn1 -- Spherical Joint 14/RConn1
  Link 18/LConn1 -- Spherical Joint 18/RConn1
  Link 12/LConn1 -- Spherical Joint 12/RConn1
  Link 2/LConn1 -- Spherical Joint 2/RConn1
  Link 1/LConn1 -- Spherical Joint 1/RConn1
  Link 13/LConn1 -- Spherical Joint 13/RConn1
  Link 5/LConn1 -- Spherical Joint 5/RConn1
  Link 16/LConn1 -- Spherical Joint 16/RConn1
  Link 4/LConn1 -- Spherical Joint 4/RConn1
  Link 11/LConn1 -- Spherical Joint 11/RConn1
  Link 7/LConn1 -- Spherical Joint 7/RConn1
  Link 17/LConn1 -- Spherical Joint 17/RConn1
  Link 8/LConn1 -- Spherical Joint 8/RConn1
  Payload/RConn1 -- Angle sensor 20/LConn2 -- Link 20_last_link/RConn1 -- Transform Sensor1/RConn1 -- Angle sensor 21/LConn2 -- External Force and Torque/RConn1 -- Transform Sensor2/RConn1 -- Rigid Transform1/RConn1
  World Frame/RConn1 -- Transform Sensor1/LConn1
  PS-Simulink Converter/LConn1 -- Transform Sensor1/RConn2
  PS-Simulink Converter1/LConn1 -- Transform Sensor1/RConn3
  Unbalanced Payload/RConn1 -- Link 20_last_link1/RConn1
  Link 20_last_link1/LConn1 -- Rigid Transform2/LConn1
  Rigid Transform2/RConn1 -- Rigid Transform1/LConn1
  World Frame1/RConn1 -- Transform Sensor2/LConn1
  Transform Sensor2/RConn2 -- PS-Simulink Converter2/LConn1
  External Force and Torque/LConn1 -- Simulink-PS Converter/RConn1
  External Force and Torque/LConn2 -- Simulink-PS Converter1/RConn1

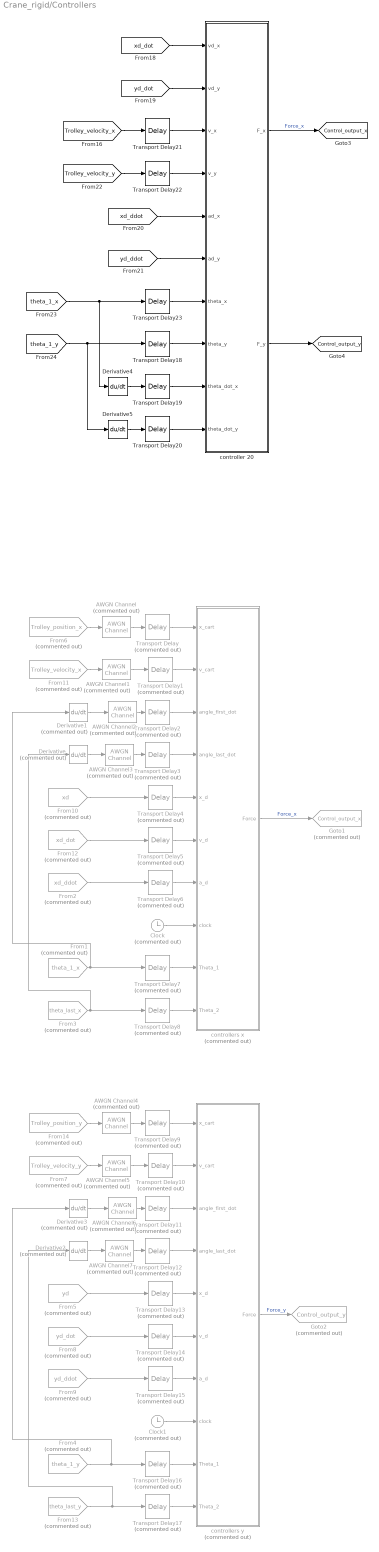
== system Crane_rigid/Controllers ==
  AWGN Channel{,1..7} (8 alike) : commchan3/AWGN Channel  Commented=on  InputProcessing=Columns as channels (frame based)  seed=67  noiseMode="Signal to noise ratio  (SNR)"  EbNodB=10  EsNodB=10  SNRdB=SNR_value  bitsPerSym=1  Ps=1  Tsym=1  variance=1
  Clock : Clock  Commented=on
  Clock1 : Clock  Commented=on
  Derivative{,1..3} (4 alike) : Derivative  Commented=on
  Derivative4 : Derivative
  Derivative5 : Derivative
  From1 : From  Commented=on  GotoTag=theta_1_x  TagVisibility=global
  From10 : From  Commented=on  GotoTag=xd  TagVisibility=global
  From11 : From  Commented=on  GotoTag=Trolley_velocity_x  TagVisibility=global
  From12 : From  Commented=on  GotoTag=xd_dot  TagVisibility=global
  From13 : From  Commented=on  GotoTag=theta_last_y  TagVisibility=global
  From14 : From  Commented=on  GotoTag=Trolley_position_y  TagVisibility=global
  From2 : From  Commented=on  GotoTag=xd_ddot  TagVisibility=global
  From3 : From  Commented=on  GotoTag=theta_last_x  TagVisibility=global
  From4 : From  Commented=on  GotoTag=theta_1_y  TagVisibility=global
  From5 : From  Commented=on  GotoTag=yd  TagVisibility=global
  From6 : From  Commented=on  GotoTag=Trolley_position_x  TagVisibility=global
  From7 : From  Commented=on  GotoTag=Trolley_velocity_y  TagVisibility=global
  From8 : From  Commented=on  GotoTag=yd_dot  TagVisibility=global
  From9 : From  Commented=on  GotoTag=yd_ddot  TagVisibility=global
  Goto1 : Goto  Commented=on  GotoTag=Control_output_x  TagVisibility=global
  Goto2 : Goto  Commented=on  GotoTag=Control_output_y  TagVisibility=global
  Transport Delay{,1..8} (9 alike) : TransportDelay  Commented=on  DelayTime=delay_time  BufferSize=8192
  Transport Delay{9..17} (9 alike) : TransportDelay  Commented=on  DelayTime=delay_time
  Transport Delay{18..23} (6 alike) : TransportDelay  DelayTime=delay_time  BufferSize=8192
  controller 20 : Subsystem  TreatAsAtomicUnit=on  SystemSampleTime=h
  controllers x : Subsystem  Commented=on  TreatAsAtomicUnit=on  SystemSampleTime=h
  controllers y : Subsystem  Commented=on  TreatAsAtomicUnit=on  SystemSampleTime=h
  tag scope: Control_output_x=global, Control_output_y=global
  wires:
  AWGN Channel4/1 -> Transport Delay9/1
  Transport Delay10/1 -> controllers y/2(v_cart)
  AWGN Channel2/1 -> Transport Delay2/1
  Derivative1/1 -> AWGN Channel2/1
  From13/1 -> Transport Delay17/1, Derivative2/1
  Clock/1 -> controllers x/8(clock)
  From1/1 -> Transport Delay7/1, Derivative1/1
  Transport Delay13/1 -> controllers y/5(x_d)
  Transport Delay1/1 -> controllers x/2(v_cart)
  AWGN Channel6/1 -> Transport Delay11/1
  Derivative/1 -> AWGN Channel3/1
  Transport Delay8/1 -> controllers x/10(Theta_2)
  Transport Delay3/1 -> controllers x/4(angle_last_dot)
  Transport Delay17/1 -> controllers y/10(Theta_2)
  Derivative2/1 -> AWGN Channel7/1
  AWGN Channel/1 -> Transport Delay/1
  From9/1 -> Transport Delay15/1
  From14/1 -> AWGN Channel4/1
  Transport Delay15/1 -> controllers y/7(a_d)
  Transport Delay/1 -> controllers x/1(x_cart)
  From4/1 -> Transport Delay16/1, Derivative3/1
  Transport Delay4/1 -> controllers x/5(x_d)
  AWGN Channel5/1 -> Transport Delay10/1
  Derivative3/1 -> AWGN Channel6/1
  Transport Delay5/1 -> controllers x/6(v_d)
  Transport Delay6/1 -> controllers x/7(a_d)
  From12/1 -> Transport Delay5/1
  Transport Delay16/1 -> controllers y/9(Theta_1)
  AWGN Channel7/1 -> Transport Delay12/1
  Clock1/1 -> controllers y/8(clock)
  Transport Delay9/1 -> controllers y/1(x_cart)
  AWGN Channel3/1 -> Transport Delay3/1
  From2/1 -> Transport Delay6/1
  From5/1 -> Transport Delay13/1
  From3/1 -> Transport Delay8/1, Derivative/1
  Transport Delay14/1 -> controllers y/6(v_d)
  From8/1 -> Transport Delay14/1
  Transport Delay2/1 -> controllers x/3(angle_first_dot)
  From7/1 -> AWGN Channel5/1
  Transport Delay11/1 -> controllers y/3(angle_first_dot)
  Transport Delay12/1 -> controllers y/4(angle_last_dot)
  AWGN Channel1/1 -> Transport Delay1/1
  From11/1 -> AWGN Channel1/1
  Transport Delay7/1 -> controllers x/9(Theta_1)
  controllers y/1(Force) -> Goto2/1  "Force_y"
  From6/1 -> AWGN Channel/1
  controllers x/1(Force) -> Goto1/1  "Force_x"
  From10/1 -> Transport Delay4/1
  [yd_ddot] -> controller 20/6(ad_y)
  controller 20/1(F_x) -> [Control_output_x]  "Force_x"
  [xd_ddot] -> controller 20/5(ad_x)
  Transport Delay23/1 -> controller 20/7(theta_x)
  Transport Delay19/1 -> controller 20/9(theta_dot_x)
  Transport Delay18/1 -> controller 20/8(theta_y)
  controller 20/2(F_y) -> [Control_output_y]
  Transport Delay20/1 -> controller 20/10(theta_dot_y)
  [theta_1_y] -> Derivative5/1, Transport Delay18/1
  Derivative5/1 -> Transport Delay20/1
  [xd_dot] -> controller 20/1(vd_x)
  [Trolley_velocity_y] -> Transport Delay22/1
  [yd_dot] -> controller 20/2(vd_y)
  Transport Delay21/1 -> controller 20/3(v_x)
  Transport Delay22/1 -> controller 20/4(v_y)
  [theta_1_x] -> Derivative4/1, Transport Delay23/1
  Derivative4/1 -> Transport Delay19/1
  [Trolley_velocity_x] -> Transport Delay21/1

== system Crane_rigid/Objectives ==
  To Workspace : ToWorkspace  VariableName=F_x_after_sat  SampleTime=h
  To Workspace1 : ToWorkspace  VariableName=F_y_after_sat  SampleTime=h
  To Workspace2 : ToWorkspace  VariableName=Trolley_position_x  SampleTime=h
  To Workspace3 : ToWorkspace  VariableName=Payload_x  SampleTime=h
  To Workspace4 : ToWorkspace  VariableName=Payload_y  SampleTime=h
  To Workspace5 : ToWorkspace  VariableName=xd  SampleTime=h
  To Workspace6 : ToWorkspace  VariableName=yd  SampleTime=h
  To Workspace7 : ToWorkspace  VariableName=Trolley_position_y  SampleTime=h
  To Workspace8 : ToWorkspace  VariableName=Payload_total_rot  SampleTime=h
  wires:
  [F_x_after_sat] -> To Workspace/1
  [F_y_after_sat] -> To Workspace1/1
  [Trolley_position_x] -> To Workspace2/1
  [Payload_x] -> To Workspace3/1
  [Payload_y] -> To Workspace4/1
  [xd] -> To Workspace5/1
  [yd] -> To Workspace6/1
  [Trolley_position_y] -> To Workspace7/1
  [Payload_total_rot] -> To Workspace8/1
